simulink model "Lab05Exp"  (Simulink 7.1)
settings: Solver=ode45  StartTime=0.0  StopTime=20  RelTol=1e-3
settings Model: Creator=George  LastModifiedBy=George

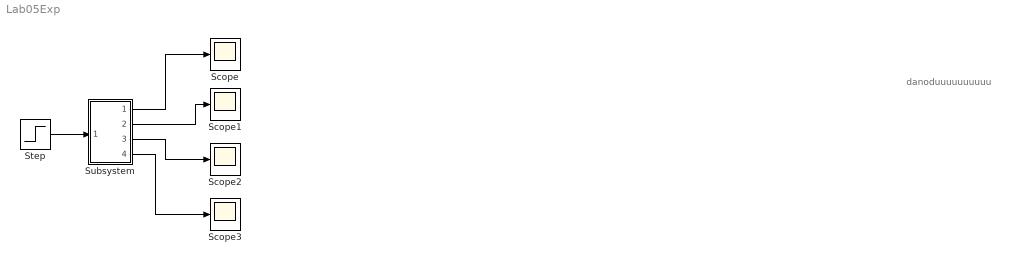
== system Lab05Exp ==
  note: danoduuuuuuuuuu
  Scope{,1..3} (4 alike) : Scope
      Scope2 settings: SaveName=ScopeData2
      Scope3 settings: SaveName=ScopeData3
  Step : Step  After=0  SampleTime=0
  Subsystem : Subsystem  mask{M=2, mp=0.25, L=0.4, B=0.2, g=9.8}
  wires:
  Step/1 -> Subsystem/1(In1)
  Subsystem/1(Out1) -> Scope/1
  Subsystem/2(Out2) -> Scope1/1
  Subsystem/3(Out3) -> Scope2/1
  Subsystem/4(Out4) -> Scope3/1

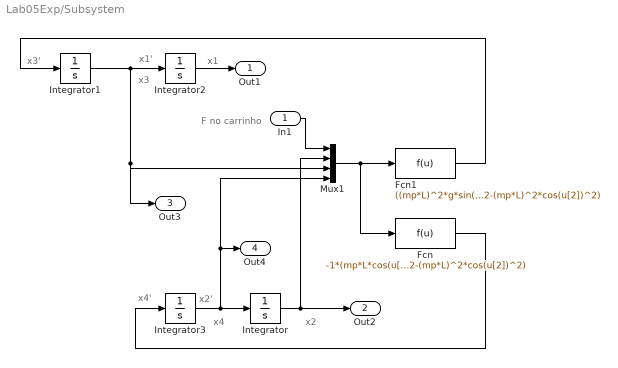
== system Lab05Exp/Subsystem ==
  note: F no carrinho
  note: x2'
  note: x1'
  note: x2
  note: x4
  note: x4'
  note: x1
  note: x3
  note: x3'
  In1 : Inport  OutDataType=sfix(16)  OutScaling=2^0
  Fcn : Fcn  Expr=-1*(mp*L*cos(u[2])*(-1*B*u[3]+mp*L*u[4]^2*sin(u[2])+u[1])+(M+mp)*mp*g*L*sin(u[2]))/((M+mp)*4/3*mp*L^2-(mp*L)^2*cos(u[2])^2)
  Fcn1 : Fcn  Expr=((mp*L)^2*g*sin(u[2])*cos(u[2])+4/3*mp*L^2*(-1*B*u[3]+mp*L*u[4]^2*sin(u[2])+u[1]))/((M+mp)*4/3*mp*L^2-(mp*L)^2*cos(u[2])^2)
  Integrator : Integrator  InitialCondition=pi/3
  Integrator1 : Integrator
  Integrator2 : Integrator
  Integrator3 : Integrator
  Mux1 : Mux
  Out1 : Outport  OutDataType=sfix(16)  OutScaling=2^0
  Out2 : Outport  Port=2  OutDataType=sfix(16)  OutScaling=2^0
  Out3 : Outport  Port=3  OutDataType=sfix(16)  OutScaling=2^0
  Out4 : Outport  Port=4  OutDataType=sfix(16)  OutScaling=2^0
  wires:
  Integrator/1 -> Mux1/2, Out2/1
  Integrator3/1 -> Integrator/1, Mux1/4, Out4/1
  Fcn/1 -> Integrator3/1
  Integrator2/1 -> Out1/1
  Integrator1/1 -> Integrator2/1, Mux1/3, Out3/1
  Fcn1/1 -> Integrator1/1
  Mux1/1 -> Fcn1/1, Fcn/1
  In1/1 -> Mux1/1
